simulink model "reftracking_LinearTopTest"  (R2018a)
settings: Solver=ode15s  StartTime=0.0  StopTime=10  FixedStep=h  RelTol=1e-3
values from neighbouring files (symbols this model uses):
  Parameters = CoenParams(X)    [EstimatedParams.m]    (also in LQR.m = EstimatedParams(); LSQnonLinfunc.m; TestModel.m = CoenParams(X0); testingLQRDisturbance.m = EstimatedParams())
settings Model: PauseTimes=1  Creator=coeng  LastModifiedBy=BozeMannen
settings DataIOCC: ReturnWorkspaceOutputs=on
settings DebuggingCC: ModelReferenceExtraNoncontSigs=warning
settings SFSimCC: SimUseLocalCustomCode=on
settings RTWCC: RTWUseLocalCustomCode=on
settings CodeAppCC: StateflowObjectComments=on

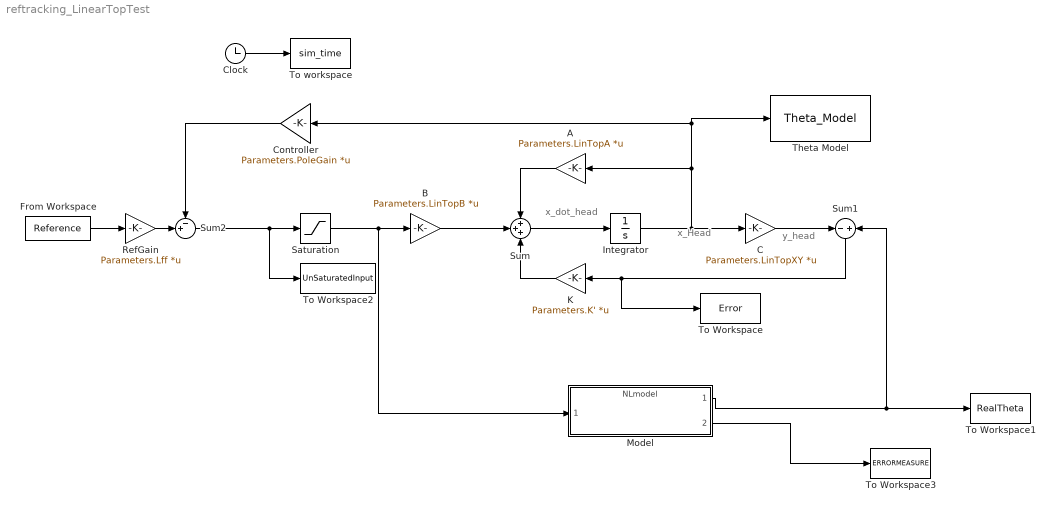
== system reftracking_LinearTopTest ==
  note: y_head
  note: x_dot_head
  note: x_Head
  A : Gain  Gain=Parameters.LinTopA  Multiplication=Matrix(K*u)
  B : Gain  Gain=Parameters.LinTopB  Multiplication=Matrix(K*u)
  C : Gain  Gain=Parameters.LinTopXY  Multiplication=Matrix(K*u)
  Clock : Clock
  Controller : Gain  Gain=Parameters.PoleGain  Multiplication=Matrix(K*u)
  From Workspace : FromWorkspace  VariableName=Reference  SampleTime=0
  Integrator : Integrator  InitialCondition=firstLocationFull'
  K : Gain  Gain=Parameters.K'  Multiplication=Matrix(K*u)
  Model : ModelReference  ModelNameDialog=NLmodel  SimulationMode=Normal  ModelReferenceVersion=1.108
  RefGain : Gain  Gain=Parameters.Lff  Multiplication=Matrix(K*u)
  Saturation : Saturate
  Sum : Sum  Inputs=+++
  Sum1 : Sum  Inputs=-|+
  Sum2 : Sum  Inputs=-+|
  Theta Model : ToWorkspace  VariableName=Theta_Model  SaveFormat=Timeseries  SampleTime=-1
  To Workspace : ToWorkspace  VariableName=Error  SaveFormat=Timeseries  SampleTime=-1
  To Workspace1 : ToWorkspace  VariableName=RealTheta  SaveFormat=Timeseries  SampleTime=-1
  To Workspace2 : ToWorkspace  VariableName=UnSaturatedInput  SaveFormat=Timeseries  SampleTime=-1
  To Workspace3 : ToWorkspace  VariableName=ERRORMEASURE  SaveFormat=Timeseries  SampleTime=-1
  To workspace : ToWorkspace  VariableName=sim_time  SaveFormat=Timeseries  SampleTime=-1
  wires:
  Sum/1 -> Integrator/1
  Integrator/1 -> C/1, A/1, Controller/1, Theta Model/1
  Sum1/1 -> K/1, To Workspace/1
  C/1 -> Sum1/1
  Controller/1 -> Sum2/1
  A/1 -> Sum/1
  B/1 -> Sum/2
  Model/1 -> Sum1/2, To Workspace1/1
  K/1 -> Sum/3
  Sum2/1 -> Saturation/1, To Workspace2/1
  Saturation/1 -> Model/1, B/1
  Model/2 -> To Workspace3/1
  From Workspace/1 -> RefGain/1
  RefGain/1 -> Sum2/2
  Clock/1 -> To workspace/1
